simulink model "VehicleModel_Connected"  (R2025a)
settings: Solver=VariableStepAuto  StartTime=0.0  StopTime=10.0  RelTol=1e-3
libraries: autosarlibfim x1, sldvlib x1
settings Model: Creator=uss924001  LastModifiedBy=uss924001

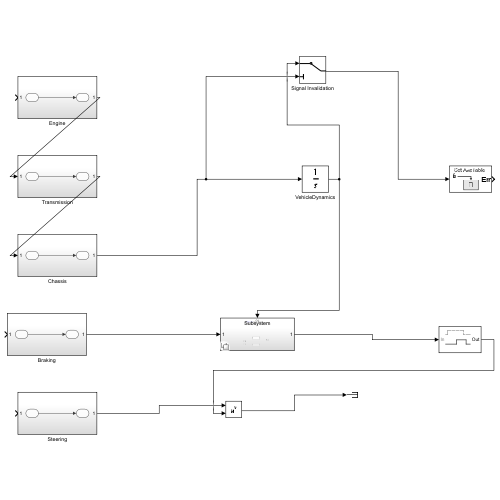
[thumbnail: Simulink's stored preview of the top-level diagram]
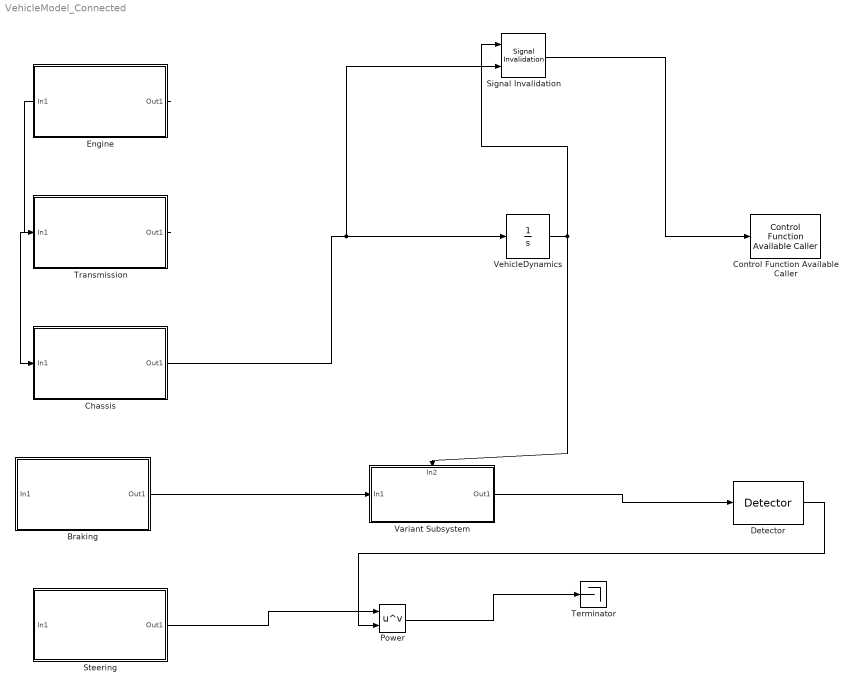
== system VehicleModel_Connected ==
  Braking : Subsystem
  Chassis : Subsystem
  Control Function Available Caller : autosarlibfim/Control Function Available Caller  PortName=ControlFunctionAvailable  Operation=SetFunctionAvailable  st=-1  ServiceImpl=autosar.bsw.FiM_ControlFunctionAvailable  SyncToSchema=off  FunctionPrototypeCache=ERR = ControlFunctionAvailable_SetFunctionAvailable(Availability)
  Detector : sldvlib/Temporal Operators/Detector  reset=off  typ=Delayed Fixed Duration  in_hold=2  delay=1  out_hold=3
  Engine : Subsystem
  Power : Math  Operator=pow
  Signal Invalidation : SignalInvalidation
  Steering : Subsystem
  Terminator : Terminator
  Transmission : Subsystem
  Variant Subsystem : Subsystem  Variant=on
      settings: PortSchema="{\"entries\":[{\"content\":{\"sides\":[{\"content\":{\"connectorIds\":[\"In1\"]},\"type\":\"ConnectorPlacement.EquallySpacedRectSide\",\"uuid\":\"68b98c4a-1491-4a6c-a325-756e56336f12\"},{\"content\":{\"connectorIds\":[\"Out1\"],\"side\":\"RIGHT\"},\"type\":\"ConnectorPlacement.EquallySpacedRectSide\",\"uuid\":\"87cc84e8-6904-4545-b329-5179fc83f7d1\"},{\"content\":{\"connectorIds\":[\"In2\"],\"side\":\"TOP\"},\"type\":\"ConnectorPlacement.EquallySpacedRectSide\",\"uuid\":\"b3ee15ed-d029-49c7-90d5-9fcbcca69a59\"}]},\"type\":\"ConnectorPlacement.EquallySpacedConnector\",\"uuid\":\"9accc581-43a0-4513-a532-03ae5f42fb51\"}],\"packageUris\":[\"http://schema.mathworks.com/mf0/Connector/R2020b\"],\"version\":\"1.0\"}"
  VehicleDynamics : Integrator
  wires:
  Engine/1(Out1) -> Transmission/1(In1)
  Transmission/1(Out1) -> Chassis/1(In1)
  Braking/1(Out1) -> Variant Subsystem/1(In1)
  VehicleDynamics/1 -> Signal Invalidation/1, Variant Subsystem/2(In2)
  Chassis/1(Out1) -> Signal Invalidation/2, VehicleDynamics/1
  Signal Invalidation/1 -> Control Function Available Caller/1
  Variant Subsystem/1(Out1) -> Detector/1
  Steering/1(Out1) -> Power/1
  Power/1 -> Terminator/1
  Detector/1 -> Power/2

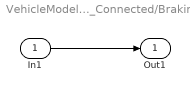
== system VehicleModel_Connected/Braking ==
  In1 : Inport
  Out1 : Outport
  wires:
  In1/1 -> Out1/1

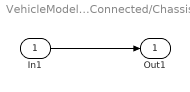
== system VehicleModel_Connected/Chassis ==
  In1 : Inport
  Out1 : Outport
  wires:
  In1/1 -> Out1/1

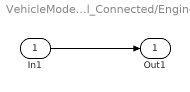
== system VehicleModel_Connected/Engine ==
  In1 : Inport
  Out1 : Outport
  wires:
  In1/1 -> Out1/1

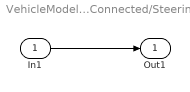
== system VehicleModel_Connected/Steering ==
  In1 : Inport
  Out1 : Outport
  wires:
  In1/1 -> Out1/1

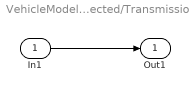
== system VehicleModel_Connected/Transmission ==
  In1 : Inport
  Out1 : Outport
  wires:
  In1/1 -> Out1/1

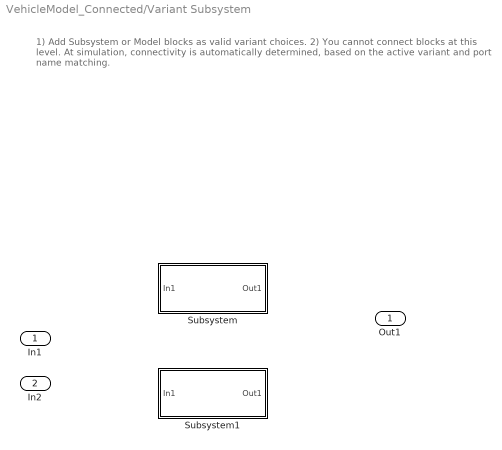
== system VehicleModel_Connected/Variant Subsystem ==
  note: 1) Add Subsystem or Model blocks as valid variant choices.
      | 2) You cannot connect blocks at this level. At simulation, connectivity is automatically
      | determined, based on the active variant and port name matching.
  In1 : Inport
  In2 : Inport  Port=2
  Subsystem : Subsystem  VariantControl=true
  Subsystem1 : Subsystem  VariantControl=false
  Out1 : Outport

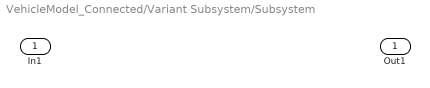
== system VehicleModel_Connected/Variant Subsystem/Subsystem ==
  In1 : Inport
  Out1 : Outport

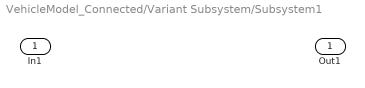
== system VehicleModel_Connected/Variant Subsystem/Subsystem1 ==
  In1 : Inport
  Out1 : Outport
